simulink model "pitch_damper"  (R2018a)
settings: Solver=VariableStepAuto  StartTime=0.0  StopTime=10.0  RelTol=1e-3
values from neighbouring files (symbols this model uses):
  A = [xu xa xt 0    xug                  xag       0 ... (first row only)    [cit2s.m]    (also in dumfile.mat = [-0.0363411031287 -0.37648768923 0 0.00913670110478 0 0 0 0.; dumpfile.mat = [-0.143125941665 0 -0.415614299261 0.297675031169 0 0 0 0 0 ; main.m = A-B(:,1)*K; main_old.m = [xu xa xt 0    xug                  xag       0 0)
  B = [xd 0                                 0 ... (first row only)    [cit2s.m]    (also in dumfile.mat = [0 -0.103368406929 0 -0.262514547046 0 0 0 0 0 0 0 0.0050931; dumpfile.mat = [0 0 -1.41903488661 -0.0208070113439 0 0 0 0 0 0 0.043924159; main.m; main_old.m)
  C = eye ( 7 )    [cit2s.m]    (also in main.m = [eye(4) zeros(4,3); main_old.m = eye (8))
  D = zeros ( 7 , 3 )    [cit2s.m]    (also in main.m = [zeros(4,3); main_old.m = zeros (8 , 3 ))
  K = [0 0 Kt Kq 0 0 0]    [cit2s.m]    (also in main.m = [0 Ka Kt Kq 0 0 0 ]; main_old.m = [0 Ka Kt Kq 0 0 0 0])
settings Model: Creator=bart  LastModifiedBy=bart

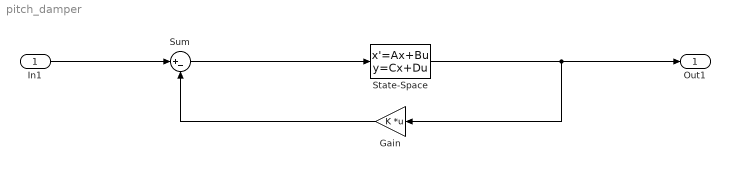
== system pitch_damper ==
  In1 : Inport
  Gain : Gain  Gain=K  Multiplication=Matrix(K*u)
  State-Space : StateSpace  A=A  B=B  C=C  D=D  InitialCondition=0
  Sum : Sum  Inputs=|+-
  Out1 : Outport
  wires:
  Sum/1 -> State-Space/1
  State-Space/1 -> Gain/1, Out1/1
  In1/1 -> Sum/1
  Gain/1 -> Sum/2
